simulink model "Dynamics"  (R2015a)
settings: Solver=ode45  StartTime=0.0  StopTime=50  FixedStep=1e-3
libraries: aerolibutil x16, aerolibtransform2 x6, dspmtrx3 x6
(part 2 of 2)

== system Dynamics/Jacobian/J_v/J_v_3 ==
  R : Inport
  p : Inport  Port=2
  pn : Inport  Port=3
  type : Inport  Port=4
  Add : Sum
  If : If  IfExpression=u1 == 1
  Prismatic Action : Subsystem  TreatAsAtomicUnit=on
  Revolute Action : Subsystem  TreatAsAtomicUnit=on
  J_v : Outport
  wires:
  type/1 -> If/1
  If/1 -> Revolute Action/Action
  If/2 -> Prismatic Action/Action
  Revolute Action/1(J_v) -> Add/1
  Prismatic Action/1(J_v) -> Add/2
  Add/1 -> J_v/1
  R/1 -> Prismatic Action/1(R), Revolute Action/1(R)
  p/1 -> Revolute Action/2(p)
  pn/1 -> Revolute Action/3(pn)

== system Dynamics/Jacobian/J_v/J_v_4 ==
  R : Inport
  p : Inport  Port=2
  pn : Inport  Port=3
  type : Inport  Port=4
  Add : Sum
  If : If  IfExpression=u1 == 1
  Prismatic Action : Subsystem  TreatAsAtomicUnit=on
  Revolute Action : Subsystem  TreatAsAtomicUnit=on
  J_v : Outport
  wires:
  type/1 -> If/1
  If/1 -> Revolute Action/Action
  If/2 -> Prismatic Action/Action
  Revolute Action/1(J_v) -> Add/1
  Prismatic Action/1(J_v) -> Add/2
  Add/1 -> J_v/1
  R/1 -> Prismatic Action/1(R), Revolute Action/1(R)
  p/1 -> Revolute Action/2(p)
  pn/1 -> Revolute Action/3(pn)

== system Dynamics/Jacobian/J_v/J_v_5 ==
  R : Inport
  p : Inport  Port=2
  pn : Inport  Port=3
  type : Inport  Port=4
  Add : Sum
  If : If  IfExpression=u1 == 1
  Prismatic Action : Subsystem  TreatAsAtomicUnit=on
  Revolute Action : Subsystem  TreatAsAtomicUnit=on
  J_v : Outport
  wires:
  type/1 -> If/1
  If/1 -> Revolute Action/Action
  If/2 -> Prismatic Action/Action
  Revolute Action/1(J_v) -> Add/1
  Prismatic Action/1(J_v) -> Add/2
  Add/1 -> J_v/1
  R/1 -> Prismatic Action/1(R), Revolute Action/1(R)
  p/1 -> Revolute Action/2(p)
  pn/1 -> Revolute Action/3(pn)

== system Dynamics/Jacobian/J_v/J_v_6 ==
  R : Inport
  p : Inport  Port=2
  pn : Inport  Port=3
  type : Inport  Port=4
  Add : Sum
  If : If  IfExpression=u1 == 1
  Prismatic Action : Subsystem  TreatAsAtomicUnit=on
  Revolute Action : Subsystem  TreatAsAtomicUnit=on
  J_v : Outport
  wires:
  type/1 -> If/1
  If/1 -> Revolute Action/Action
  If/2 -> Prismatic Action/Action
  Revolute Action/1(J_v) -> Add/1
  Prismatic Action/1(J_v) -> Add/2
  Add/1 -> J_v/1
  R/1 -> Prismatic Action/1(R), Revolute Action/1(R)
  p/1 -> Revolute Action/2(p)
  pn/1 -> Revolute Action/3(pn)

== system Dynamics/Jacobian/J(q) gen./J_v_2(q)/J_v_1 ==
  R : Inport
  p : Inport  Port=2
  pn : Inport  Port=3
  type : Inport  Port=4
  Add : Sum
  If : If  IfExpression=u1 == 1
  Prismatic Action : Subsystem  TreatAsAtomicUnit=on
  Revolute Action : Subsystem  TreatAsAtomicUnit=on
  J_v : Outport
  wires:
  type/1 -> If/1
  If/1 -> Revolute Action/Action
  If/2 -> Prismatic Action/Action
  Revolute Action/1(J_v) -> Add/1
  Prismatic Action/1(J_v) -> Add/2
  Add/1 -> J_v/1
  R/1 -> Prismatic Action/1(R), Revolute Action/1(R)
  p/1 -> Revolute Action/2(p)
  pn/1 -> Revolute Action/3(pn)

== system Dynamics/Jacobian/J(q) gen./J_v_3(q)/J_v_1 ==
  R : Inport
  p : Inport  Port=2
  pn : Inport  Port=3
  type : Inport  Port=4
  Add : Sum
  If : If  IfExpression=u1 == 1
  Prismatic Action : Subsystem  TreatAsAtomicUnit=on
  Revolute Action : Subsystem  TreatAsAtomicUnit=on
  J_v : Outport
  wires:
  type/1 -> If/1
  If/1 -> Revolute Action/Action
  If/2 -> Prismatic Action/Action
  Revolute Action/1(J_v) -> Add/1
  Prismatic Action/1(J_v) -> Add/2
  Add/1 -> J_v/1
  R/1 -> Prismatic Action/1(R), Revolute Action/1(R)
  p/1 -> Revolute Action/2(p)
  pn/1 -> Revolute Action/3(pn)

== system Dynamics/Jacobian/J(q) gen./J_v_3(q)/J_v_2 ==
  R : Inport
  p : Inport  Port=2
  pn : Inport  Port=3
  type : Inport  Port=4
  Add : Sum
  If : If  IfExpression=u1 == 1
  Prismatic Action : Subsystem  TreatAsAtomicUnit=on
  Revolute Action : Subsystem  TreatAsAtomicUnit=on
  J_v : Outport
  wires:
  type/1 -> If/1
  If/1 -> Revolute Action/Action
  If/2 -> Prismatic Action/Action
  Revolute Action/1(J_v) -> Add/1
  Prismatic Action/1(J_v) -> Add/2
  Add/1 -> J_v/1
  R/1 -> Prismatic Action/1(R), Revolute Action/1(R)
  p/1 -> Revolute Action/2(p)
  pn/1 -> Revolute Action/3(pn)

== system Dynamics/Jacobian/J(q) gen./J_v_4(q)/J_v_1 ==
  R : Inport
  p : Inport  Port=2
  pn : Inport  Port=3
  type : Inport  Port=4
  Add : Sum
  If : If  IfExpression=u1 == 1
  Prismatic Action : Subsystem  TreatAsAtomicUnit=on
  Revolute Action : Subsystem  TreatAsAtomicUnit=on
  J_v : Outport
  wires:
  type/1 -> If/1
  If/1 -> Revolute Action/Action
  If/2 -> Prismatic Action/Action
  Revolute Action/1(J_v) -> Add/1
  Prismatic Action/1(J_v) -> Add/2
  Add/1 -> J_v/1
  R/1 -> Prismatic Action/1(R), Revolute Action/1(R)
  p/1 -> Revolute Action/2(p)
  pn/1 -> Revolute Action/3(pn)

== system Dynamics/Jacobian/J(q) gen./J_v_4(q)/J_v_2 ==
  R : Inport
  p : Inport  Port=2
  pn : Inport  Port=3
  type : Inport  Port=4
  Add : Sum
  If : If  IfExpression=u1 == 1
  Prismatic Action : Subsystem  TreatAsAtomicUnit=on
  Revolute Action : Subsystem  TreatAsAtomicUnit=on
  J_v : Outport
  wires:
  type/1 -> If/1
  If/1 -> Revolute Action/Action
  If/2 -> Prismatic Action/Action
  Revolute Action/1(J_v) -> Add/1
  Prismatic Action/1(J_v) -> Add/2
  Add/1 -> J_v/1
  R/1 -> Prismatic Action/1(R), Revolute Action/1(R)
  p/1 -> Revolute Action/2(p)
  pn/1 -> Revolute Action/3(pn)

== system Dynamics/Jacobian/J(q) gen./J_v_4(q)/J_v_3 ==
  R : Inport
  p : Inport  Port=2
  pn : Inport  Port=3
  type : Inport  Port=4
  Add : Sum
  If : If  IfExpression=u1 == 1
  Prismatic Action : Subsystem  TreatAsAtomicUnit=on
  Revolute Action : Subsystem  TreatAsAtomicUnit=on
  J_v : Outport
  wires:
  type/1 -> If/1
  If/1 -> Revolute Action/Action
  If/2 -> Prismatic Action/Action
  Revolute Action/1(J_v) -> Add/1
  Prismatic Action/1(J_v) -> Add/2
  Add/1 -> J_v/1
  R/1 -> Prismatic Action/1(R), Revolute Action/1(R)
  p/1 -> Revolute Action/2(p)
  pn/1 -> Revolute Action/3(pn)

== system Dynamics/Jacobian/J(q) gen./J_v_5(q)/J_v_1 ==
  R : Inport
  p : Inport  Port=2
  pn : Inport  Port=3
  type : Inport  Port=4
  Add : Sum
  If : If  IfExpression=u1 == 1
  Prismatic Action : Subsystem  TreatAsAtomicUnit=on
  Revolute Action : Subsystem  TreatAsAtomicUnit=on
  J_v : Outport
  wires:
  type/1 -> If/1
  If/1 -> Revolute Action/Action
  If/2 -> Prismatic Action/Action
  Revolute Action/1(J_v) -> Add/1
  Prismatic Action/1(J_v) -> Add/2
  Add/1 -> J_v/1
  R/1 -> Prismatic Action/1(R), Revolute Action/1(R)
  p/1 -> Revolute Action/2(p)
  pn/1 -> Revolute Action/3(pn)

== system Dynamics/Jacobian/J(q) gen./J_v_5(q)/J_v_2 ==
  R : Inport
  p : Inport  Port=2
  pn : Inport  Port=3
  type : Inport  Port=4
  Add : Sum
  If : If  IfExpression=u1 == 1
  Prismatic Action : Subsystem  TreatAsAtomicUnit=on
  Revolute Action : Subsystem  TreatAsAtomicUnit=on
  J_v : Outport
  wires:
  type/1 -> If/1
  If/1 -> Revolute Action/Action
  If/2 -> Prismatic Action/Action
  Revolute Action/1(J_v) -> Add/1
  Prismatic Action/1(J_v) -> Add/2
  Add/1 -> J_v/1
  R/1 -> Prismatic Action/1(R), Revolute Action/1(R)
  p/1 -> Revolute Action/2(p)
  pn/1 -> Revolute Action/3(pn)

== system Dynamics/Jacobian/J(q) gen./J_v_5(q)/J_v_3 ==
  R : Inport
  p : Inport  Port=2
  pn : Inport  Port=3
  type : Inport  Port=4
  Add : Sum
  If : If  IfExpression=u1 == 1
  Prismatic Action : Subsystem  TreatAsAtomicUnit=on
  Revolute Action : Subsystem  TreatAsAtomicUnit=on
  J_v : Outport
  wires:
  type/1 -> If/1
  If/1 -> Revolute Action/Action
  If/2 -> Prismatic Action/Action
  Revolute Action/1(J_v) -> Add/1
  Prismatic Action/1(J_v) -> Add/2
  Add/1 -> J_v/1
  R/1 -> Prismatic Action/1(R), Revolute Action/1(R)
  p/1 -> Revolute Action/2(p)
  pn/1 -> Revolute Action/3(pn)

== system Dynamics/Jacobian/J(q) gen./J_v_5(q)/J_v_4 ==
  R : Inport
  p : Inport  Port=2
  pn : Inport  Port=3
  type : Inport  Port=4
  Add : Sum
  If : If  IfExpression=u1 == 1
  Prismatic Action : Subsystem  TreatAsAtomicUnit=on
  Revolute Action : Subsystem  TreatAsAtomicUnit=on
  J_v : Outport
  wires:
  type/1 -> If/1
  If/1 -> Revolute Action/Action
  If/2 -> Prismatic Action/Action
  Revolute Action/1(J_v) -> Add/1
  Prismatic Action/1(J_v) -> Add/2
  Add/1 -> J_v/1
  R/1 -> Prismatic Action/1(R), Revolute Action/1(R)
  p/1 -> Revolute Action/2(p)
  pn/1 -> Revolute Action/3(pn)

== system Dynamics/Jacobian/J_v/J_v_1/Prismatic Action ==
  R : Inport
  Action Port : ActionPort  ActionType=else
  Constant : Constant  Value=[0;0;1]
  Product : Product  Multiplication=Matrix(*)
  J_v : Outport
  wires:
  Product/1 -> J_v/1
  R/1 -> Product/1
  Constant/1 -> Product/2

== system Dynamics/Jacobian/J_v/J_v_1/Revolute Action ==
  R : Inport
  p : Inport  Port=2
  pn : Inport  Port=3
  Action Port : ActionPort  ActionType=then
  3x3 Cross Product : aerolibutil/3x3 Cross Product
  Add : Sum  Inputs=-+
  Constant : Constant  Value=[0;0;1]
  Product : Product  Multiplication=Matrix(*)
  J_v : Outport
  wires:
  3x3 Cross Product/1 -> J_v/1
  p/1 -> Add/1
  pn/1 -> Add/2
  Add/1 -> 3x3 Cross Product/2
  R/1 -> Product/1
  Constant/1 -> Product/2
  Product/1 -> 3x3 Cross Product/1

== system Dynamics/Jacobian/J_v/J_v_2/Prismatic Action ==
  R : Inport
  Action Port : ActionPort  ActionType=else
  Constant : Constant  Value=[0;0;1]
  Product : Product  Multiplication=Matrix(*)
  J_v : Outport
  wires:
  Product/1 -> J_v/1
  R/1 -> Product/1
  Constant/1 -> Product/2

== system Dynamics/Jacobian/J_v/J_v_2/Revolute Action ==
  R : Inport
  p : Inport  Port=2
  pn : Inport  Port=3
  Action Port : ActionPort  ActionType=then
  3x3 Cross Product : aerolibutil/3x3 Cross Product
  Add : Sum  Inputs=-+
  Constant : Constant  Value=[0;0;1]
  Product : Product  Multiplication=Matrix(*)
  J_v : Outport
  wires:
  3x3 Cross Product/1 -> J_v/1
  p/1 -> Add/1
  pn/1 -> Add/2
  Add/1 -> 3x3 Cross Product/2
  R/1 -> Product/1
  Constant/1 -> Product/2
  Product/1 -> 3x3 Cross Product/1

== system Dynamics/Jacobian/J_v/J_v_3/Prismatic Action ==
  R : Inport
  Action Port : ActionPort  ActionType=else
  Constant : Constant  Value=[0;0;1]
  Product : Product  Multiplication=Matrix(*)
  J_v : Outport
  wires:
  Product/1 -> J_v/1
  R/1 -> Product/1
  Constant/1 -> Product/2

== system Dynamics/Jacobian/J_v/J_v_3/Revolute Action ==
  R : Inport
  p : Inport  Port=2
  pn : Inport  Port=3
  Action Port : ActionPort  ActionType=then
  3x3 Cross Product : aerolibutil/3x3 Cross Product
  Add : Sum  Inputs=-+
  Constant : Constant  Value=[0;0;1]
  Product : Product  Multiplication=Matrix(*)
  J_v : Outport
  wires:
  3x3 Cross Product/1 -> J_v/1
  p/1 -> Add/1
  pn/1 -> Add/2
  Add/1 -> 3x3 Cross Product/2
  R/1 -> Product/1
  Constant/1 -> Product/2
  Product/1 -> 3x3 Cross Product/1

== system Dynamics/Jacobian/J_v/J_v_4/Prismatic Action ==
  R : Inport
  Action Port : ActionPort  ActionType=else
  Constant : Constant  Value=[0;0;1]
  Product : Product  Multiplication=Matrix(*)
  J_v : Outport
  wires:
  Product/1 -> J_v/1
  R/1 -> Product/1
  Constant/1 -> Product/2

== system Dynamics/Jacobian/J_v/J_v_4/Revolute Action ==
  R : Inport
  p : Inport  Port=2
  pn : Inport  Port=3
  Action Port : ActionPort  ActionType=then
  3x3 Cross Product : aerolibutil/3x3 Cross Product
  Add : Sum  Inputs=-+
  Constant : Constant  Value=[0;0;1]
  Product : Product  Multiplication=Matrix(*)
  J_v : Outport
  wires:
  3x3 Cross Product/1 -> J_v/1
  p/1 -> Add/1
  pn/1 -> Add/2
  Add/1 -> 3x3 Cross Product/2
  R/1 -> Product/1
  Constant/1 -> Product/2
  Product/1 -> 3x3 Cross Product/1

== system Dynamics/Jacobian/J_v/J_v_5/Prismatic Action ==
  R : Inport
  Action Port : ActionPort  ActionType=else
  Constant : Constant  Value=[0;0;1]
  Product : Product  Multiplication=Matrix(*)
  J_v : Outport
  wires:
  Product/1 -> J_v/1
  R/1 -> Product/1
  Constant/1 -> Product/2

== system Dynamics/Jacobian/J_v/J_v_5/Revolute Action ==
  R : Inport
  p : Inport  Port=2
  pn : Inport  Port=3
  Action Port : ActionPort  ActionType=then
  3x3 Cross Product : aerolibutil/3x3 Cross Product
  Add : Sum  Inputs=-+
  Constant : Constant  Value=[0;0;1]
  Product : Product  Multiplication=Matrix(*)
  J_v : Outport
  wires:
  3x3 Cross Product/1 -> J_v/1
  p/1 -> Add/1
  pn/1 -> Add/2
  Add/1 -> 3x3 Cross Product/2
  R/1 -> Product/1
  Constant/1 -> Product/2
  Product/1 -> 3x3 Cross Product/1

== system Dynamics/Jacobian/J_v/J_v_6/Prismatic Action ==
  R : Inport
  Action Port : ActionPort  ActionType=else
  Constant : Constant  Value=[0;0;1]
  Product : Product  Multiplication=Matrix(*)
  J_v : Outport
  wires:
  Product/1 -> J_v/1
  R/1 -> Product/1
  Constant/1 -> Product/2

== system Dynamics/Jacobian/J_v/J_v_6/Revolute Action ==
  R : Inport
  p : Inport  Port=2
  pn : Inport  Port=3
  Action Port : ActionPort  ActionType=then
  3x3 Cross Product : aerolibutil/3x3 Cross Product
  Add : Sum  Inputs=-+
  Constant : Constant  Value=[0;0;1]
  Product : Product  Multiplication=Matrix(*)
  J_v : Outport
  wires:
  3x3 Cross Product/1 -> J_v/1
  p/1 -> Add/1
  pn/1 -> Add/2
  Add/1 -> 3x3 Cross Product/2
  R/1 -> Product/1
  Constant/1 -> Product/2
  Product/1 -> 3x3 Cross Product/1

== system Dynamics/Jacobian/J(q) gen./J_v_2(q)/J_v_1/Prismatic Action ==
  R : Inport
  Action Port : ActionPort  ActionType=else
  Constant : Constant  Value=[0;0;1]
  Product : Product  Multiplication=Matrix(*)
  J_v : Outport
  wires:
  Product/1 -> J_v/1
  R/1 -> Product/1
  Constant/1 -> Product/2

== system Dynamics/Jacobian/J(q) gen./J_v_2(q)/J_v_1/Revolute Action ==
  R : Inport
  p : Inport  Port=2
  pn : Inport  Port=3
  Action Port : ActionPort  ActionType=then
  3x3 Cross Product : aerolibutil/3x3 Cross Product
  Add : Sum  Inputs=-+
  Constant : Constant  Value=[0;0;1]
  Product : Product  Multiplication=Matrix(*)
  J_v : Outport
  wires:
  3x3 Cross Product/1 -> J_v/1
  p/1 -> Add/1
  pn/1 -> Add/2
  Add/1 -> 3x3 Cross Product/2
  R/1 -> Product/1
  Constant/1 -> Product/2
  Product/1 -> 3x3 Cross Product/1

== system Dynamics/Jacobian/J(q) gen./J_v_3(q)/J_v_1/Prismatic Action ==
  R : Inport
  Action Port : ActionPort  ActionType=else
  Constant : Constant  Value=[0;0;1]
  Product : Product  Multiplication=Matrix(*)
  J_v : Outport
  wires:
  Product/1 -> J_v/1
  R/1 -> Product/1
  Constant/1 -> Product/2

== system Dynamics/Jacobian/J(q) gen./J_v_3(q)/J_v_1/Revolute Action ==
  R : Inport
  p : Inport  Port=2
  pn : Inport  Port=3
  Action Port : ActionPort  ActionType=then
  3x3 Cross Product : aerolibutil/3x3 Cross Product
  Add : Sum  Inputs=-+
  Constant : Constant  Value=[0;0;1]
  Product : Product  Multiplication=Matrix(*)
  J_v : Outport
  wires:
  3x3 Cross Product/1 -> J_v/1
  p/1 -> Add/1
  pn/1 -> Add/2
  Add/1 -> 3x3 Cross Product/2
  R/1 -> Product/1
  Constant/1 -> Product/2
  Product/1 -> 3x3 Cross Product/1

== system Dynamics/Jacobian/J(q) gen./J_v_3(q)/J_v_2/Prismatic Action ==
  R : Inport
  Action Port : ActionPort  ActionType=else
  Constant : Constant  Value=[0;0;1]
  Product : Product  Multiplication=Matrix(*)
  J_v : Outport
  wires:
  Product/1 -> J_v/1
  R/1 -> Product/1
  Constant/1 -> Product/2

== system Dynamics/Jacobian/J(q) gen./J_v_3(q)/J_v_2/Revolute Action ==
  R : Inport
  p : Inport  Port=2
  pn : Inport  Port=3
  Action Port : ActionPort  ActionType=then
  3x3 Cross Product : aerolibutil/3x3 Cross Product
  Add : Sum  Inputs=-+
  Constant : Constant  Value=[0;0;1]
  Product : Product  Multiplication=Matrix(*)
  J_v : Outport
  wires:
  3x3 Cross Product/1 -> J_v/1
  p/1 -> Add/1
  pn/1 -> Add/2
  Add/1 -> 3x3 Cross Product/2
  R/1 -> Product/1
  Constant/1 -> Product/2
  Product/1 -> 3x3 Cross Product/1

== system Dynamics/Jacobian/J(q) gen./J_v_4(q)/J_v_1/Prismatic Action ==
  R : Inport
  Action Port : ActionPort  ActionType=else
  Constant : Constant  Value=[0;0;1]
  Product : Product  Multiplication=Matrix(*)
  J_v : Outport
  wires:
  Product/1 -> J_v/1
  R/1 -> Product/1
  Constant/1 -> Product/2

== system Dynamics/Jacobian/J(q) gen./J_v_4(q)/J_v_1/Revolute Action ==
  R : Inport
  p : Inport  Port=2
  pn : Inport  Port=3
  Action Port : ActionPort  ActionType=then
  3x3 Cross Product : aerolibutil/3x3 Cross Product
  Add : Sum  Inputs=-+
  Constant : Constant  Value=[0;0;1]
  Product : Product  Multiplication=Matrix(*)
  J_v : Outport
  wires:
  3x3 Cross Product/1 -> J_v/1
  p/1 -> Add/1
  pn/1 -> Add/2
  Add/1 -> 3x3 Cross Product/2
  R/1 -> Product/1
  Constant/1 -> Product/2
  Product/1 -> 3x3 Cross Product/1

== system Dynamics/Jacobian/J(q) gen./J_v_4(q)/J_v_2/Prismatic Action ==
  R : Inport
  Action Port : ActionPort  ActionType=else
  Constant : Constant  Value=[0;0;1]
  Product : Product  Multiplication=Matrix(*)
  J_v : Outport
  wires:
  Product/1 -> J_v/1
  R/1 -> Product/1
  Constant/1 -> Product/2

== system Dynamics/Jacobian/J(q) gen./J_v_4(q)/J_v_2/Revolute Action ==
  R : Inport
  p : Inport  Port=2
  pn : Inport  Port=3
  Action Port : ActionPort  ActionType=then
  3x3 Cross Product : aerolibutil/3x3 Cross Product
  Add : Sum  Inputs=-+
  Constant : Constant  Value=[0;0;1]
  Product : Product  Multiplication=Matrix(*)
  J_v : Outport
  wires:
  3x3 Cross Product/1 -> J_v/1
  p/1 -> Add/1
  pn/1 -> Add/2
  Add/1 -> 3x3 Cross Product/2
  R/1 -> Product/1
  Constant/1 -> Product/2
  Product/1 -> 3x3 Cross Product/1

== system Dynamics/Jacobian/J(q) gen./J_v_4(q)/J_v_3/Prismatic Action ==
  R : Inport
  Action Port : ActionPort  ActionType=else
  Constant : Constant  Value=[0;0;1]
  Product : Product  Multiplication=Matrix(*)
  J_v : Outport
  wires:
  Product/1 -> J_v/1
  R/1 -> Product/1
  Constant/1 -> Product/2

== system Dynamics/Jacobian/J(q) gen./J_v_4(q)/J_v_3/Revolute Action ==
  R : Inport
  p : Inport  Port=2
  pn : Inport  Port=3
  Action Port : ActionPort  ActionType=then
  3x3 Cross Product : aerolibutil/3x3 Cross Product
  Add : Sum  Inputs=-+
  Constant : Constant  Value=[0;0;1]
  Product : Product  Multiplication=Matrix(*)
  J_v : Outport
  wires:
  3x3 Cross Product/1 -> J_v/1
  p/1 -> Add/1
  pn/1 -> Add/2
  Add/1 -> 3x3 Cross Product/2
  R/1 -> Product/1
  Constant/1 -> Product/2
  Product/1 -> 3x3 Cross Product/1

== system Dynamics/Jacobian/J(q) gen./J_v_5(q)/J_v_1/Prismatic Action ==
  R : Inport
  Action Port : ActionPort  ActionType=else
  Constant : Constant  Value=[0;0;1]
  Product : Product  Multiplication=Matrix(*)
  J_v : Outport
  wires:
  Product/1 -> J_v/1
  R/1 -> Product/1
  Constant/1 -> Product/2

== system Dynamics/Jacobian/J(q) gen./J_v_5(q)/J_v_1/Revolute Action ==
  R : Inport
  p : Inport  Port=2
  pn : Inport  Port=3
  Action Port : ActionPort  ActionType=then
  3x3 Cross Product : aerolibutil/3x3 Cross Product
  Add : Sum  Inputs=-+
  Constant : Constant  Value=[0;0;1]
  Product : Product  Multiplication=Matrix(*)
  J_v : Outport
  wires:
  3x3 Cross Product/1 -> J_v/1
  p/1 -> Add/1
  pn/1 -> Add/2
  Add/1 -> 3x3 Cross Product/2
  R/1 -> Product/1
  Constant/1 -> Product/2
  Product/1 -> 3x3 Cross Product/1

== system Dynamics/Jacobian/J(q) gen./J_v_5(q)/J_v_2/Prismatic Action ==
  R : Inport
  Action Port : ActionPort  ActionType=else
  Constant : Constant  Value=[0;0;1]
  Product : Product  Multiplication=Matrix(*)
  J_v : Outport
  wires:
  Product/1 -> J_v/1
  R/1 -> Product/1
  Constant/1 -> Product/2

== system Dynamics/Jacobian/J(q) gen./J_v_5(q)/J_v_2/Revolute Action ==
  R : Inport
  p : Inport  Port=2
  pn : Inport  Port=3
  Action Port : ActionPort  ActionType=then
  3x3 Cross Product : aerolibutil/3x3 Cross Product
  Add : Sum  Inputs=-+
  Constant : Constant  Value=[0;0;1]
  Product : Product  Multiplication=Matrix(*)
  J_v : Outport
  wires:
  3x3 Cross Product/1 -> J_v/1
  p/1 -> Add/1
  pn/1 -> Add/2
  Add/1 -> 3x3 Cross Product/2
  R/1 -> Product/1
  Constant/1 -> Product/2
  Product/1 -> 3x3 Cross Product/1

== system Dynamics/Jacobian/J(q) gen./J_v_5(q)/J_v_3/Prismatic Action ==
  R : Inport
  Action Port : ActionPort  ActionType=else
  Constant : Constant  Value=[0;0;1]
  Product : Product  Multiplication=Matrix(*)
  J_v : Outport
  wires:
  Product/1 -> J_v/1
  R/1 -> Product/1
  Constant/1 -> Product/2

== system Dynamics/Jacobian/J(q) gen./J_v_5(q)/J_v_3/Revolute Action ==
  R : Inport
  p : Inport  Port=2
  pn : Inport  Port=3
  Action Port : ActionPort  ActionType=then
  3x3 Cross Product : aerolibutil/3x3 Cross Product
  Add : Sum  Inputs=-+
  Constant : Constant  Value=[0;0;1]
  Product : Product  Multiplication=Matrix(*)
  J_v : Outport
  wires:
  3x3 Cross Product/1 -> J_v/1
  p/1 -> Add/1
  pn/1 -> Add/2
  Add/1 -> 3x3 Cross Product/2
  R/1 -> Product/1
  Constant/1 -> Product/2
  Product/1 -> 3x3 Cross Product/1

== system Dynamics/Jacobian/J(q) gen./J_v_5(q)/J_v_4/Prismatic Action ==
  R : Inport
  Action Port : ActionPort  ActionType=else
  Constant : Constant  Value=[0;0;1]
  Product : Product  Multiplication=Matrix(*)
  J_v : Outport
  wires:
  Product/1 -> J_v/1
  R/1 -> Product/1
  Constant/1 -> Product/2

== system Dynamics/Jacobian/J(q) gen./J_v_5(q)/J_v_4/Revolute Action ==
  R : Inport
  p : Inport  Port=2
  pn : Inport  Port=3
  Action Port : ActionPort  ActionType=then
  3x3 Cross Product : aerolibutil/3x3 Cross Product
  Add : Sum  Inputs=-+
  Constant : Constant  Value=[0;0;1]
  Product : Product  Multiplication=Matrix(*)
  J_v : Outport
  wires:
  3x3 Cross Product/1 -> J_v/1
  p/1 -> Add/1
  pn/1 -> Add/2
  Add/1 -> 3x3 Cross Product/2
  R/1 -> Product/1
  Constant/1 -> Product/2
  Product/1 -> 3x3 Cross Product/1

== matlab function Dynamics/H_6^0/H_5^4/MATLAB Function ==
  data: R input; H output; p input
function H = fcn(R,p)

H = [R          p
     zeros(1,3) 1];

== matlab function Dynamics/H_6^0/H_4^3/MATLAB Function ==
  data: R input; H output; p input
function H = fcn(R,p)

H = [R          p
     zeros(1,3) 1];

== matlab function Dynamics/H_6^0/H_3^2/MATLAB Function ==
  data: R input; H output; p input
function H = fcn(R,p)

H = [R          p
     zeros(1,3) 1];

== matlab function Dynamics/H_6^0/H_2^1/MATLAB Function ==
  data: R input; H output; p input
function H = fcn(R,p)

H = [R          p
     zeros(1,3) 1];

== matlab function Dynamics/H_6^0/H_1^0/MATLAB Function ==
  data: R input; H output; p input
function H = fcn(R,p)

H = [R          p
     zeros(1,3) 1];

== matlab function Dynamics/Jacobian/J(q) gen./J_v_1(q)/v2M_1 ==
  data: v1 input; M output; v2 input
function M = fcn(v1,v2)

M=[v1 v2];

== matlab function Dynamics/Jacobian/J_w/J_w_1 ==
  data: R input; J_w output; type input
function J_w = fcn(R,type)

if type==1
    
    J_w=R*[0;0;1];
    
else
    
    J_w=zeros(3,1);
    
end

== matlab function Dynamics/H_6^0/H_6^5/MATLAB Function ==
  data: R input; H output; p input
function H = fcn(R,p)

H = [R          p
     zeros(1,3) 1];

== matlab function Dynamics/Jacobian/J_w/J_w_2 ==
  data: R input; J_w output; type input
function J_w = fcn(R,type)

if type==1
    
    J_w=R*[0;0;1];
    
else
    
    J_w=zeros(3,1);
    
end

== matlab function Dynamics/Jacobian/J_w/J_w_3 ==
  data: R input; J_w output; type input
function J_w = fcn(R,type)

if type==1
    
    J_w=R*[0;0;1];
    
else
    
    J_w=zeros(3,1);
    
end

== matlab function Dynamics/Jacobian/J_w/J_w_4 ==
  data: R input; J_w output; type input
function J_w = fcn(R,type)

if type==1
    
    J_w=R*[0;0;1];
    
else
    
    J_w=zeros(3,1);
    
end

== matlab function Dynamics/Jacobian/J_w/J_w_5 ==
  data: R input; J_w output; type input
function J_w = fcn(R,type)

if type==1
    
    J_w=R*[0;0;1];
    
else
    
    J_w=zeros(3,1);
    
end

== matlab function Dynamics/Jacobian/J_w/J_w_6 ==
  data: R input; J_w output; type input
function J_w = fcn(R,type)

if type==1
    
    J_w=R*[0;0;1];
    
else
    
    J_w=zeros(3,1);
    
end

== matlab function Dynamics/Jacobian/J_w/v2M_1 ==
  data: v1 input; M output; v2 input
function M = fcn(v1,v2)

M=[v1 v2];

== matlab function Dynamics/Jacobian/J_w/v2M_2 ==
  data: v1 input; M output; v2 input
function M = fcn(v1,v2)

M=[v1 v2];

== matlab function Dynamics/Jacobian/J_w/v2M_3 ==
  data: v1 input; M output; v2 input
function M = fcn(v1,v2)

M=[v1 v2];

== matlab function Dynamics/Jacobian/J_w/v2M_4 ==
  data: v1 input; M output; v2 input
function M = fcn(v1,v2)

M=[v1 v2];

== matlab function Dynamics/Jacobian/J_w/v2M_5 ==
  data: v1 input; M output; v2 input
function M = fcn(v1,v2)

M=[v1 v2];

== matlab function Dynamics/Jacobian/J(q) gen./J_v_1(q)/v2M_2 ==
  data: v1 input; M output; v2 input
function M = fcn(v1,v2)

M=[v1 v2];

== matlab function Dynamics/Jacobian/J(q) gen./J_v_1(q)/v2M_3 ==
  data: v1 input; M output; v2 input
function M = fcn(v1,v2)

M=[v1 v2];

== matlab function Dynamics/Jacobian/J(q) gen./J_v_1(q)/v2M_4 ==
  data: v1 input; M output; v2 input
function M = fcn(v1,v2)

M=[v1 v2];

== matlab function Dynamics/Jacobian/J(q) gen./J_v_1(q)/v2M_5 ==
  data: v1 input; M output; v2 input
function M = fcn(v1,v2)

M=[v1 v2];

== matlab function Dynamics/Jacobian/J(q) gen./J_v_2(q)/v2M_1 ==
  data: v1 input; M output; v2 input
function M = fcn(v1,v2)

M=[v1 v2];

== matlab function Dynamics/Jacobian/J(q) gen./J_v_2(q)/v2M_2 ==
  data: v1 input; M output; v2 input
function M = fcn(v1,v2)

M=[v1 v2];

== matlab function Dynamics/Jacobian/J_v/v2M_1 ==
  data: v1 input; M output; v2 input
function M = fcn(v1,v2)

M=[v1 v2];

== matlab function Dynamics/Jacobian/J_v/v2M_2 ==
  data: v1 input; M output; v2 input
function M = fcn(v1,v2)

M=[v1 v2];

== matlab function Dynamics/Jacobian/J_v/v2M_3 ==
  data: v1 input; M output; v2 input
function M = fcn(v1,v2)

M=[v1 v2];

== matlab function Dynamics/Jacobian/J_v/v2M_4 ==
  data: v1 input; M output; v2 input
function M = fcn(v1,v2)

M=[v1 v2];

== matlab function Dynamics/Jacobian/J_v/v2M_5 ==
  data: v1 input; M output; v2 input
function M = fcn(v1,v2)

M=[v1 v2];

== matlab function Dynamics/M(q),C(q,dq),g(q)/M,H/MATLAB Function ==
  data: m input; M output; I1 input; I2 input; I3 input; I4 input; I5 input; I6 input; W1 input; W2 input; W3 input; W4 input; W5 input; W6 input; H output
function [M,H] = fcn(m,I1,I2,I3,I4,I5,I6,W1,W2,W3,W4,W5,W6)
%#codegen

M = blkdiag(m(1)*eye(3),m(2)*eye(3),m(3)*eye(3),m(4)*eye(3),m(5)*eye(3),m(6)*eye(3),...
            I1,I2,I3,I4,I5,I6);

H =-blkdiag(zeros(18,18),W1,W2,W3,W4,W5,W6);

== matlab function Dynamics/M(q),C(q,dq),g(q)/M,H/W1 ==
  data: w1 input; W output; w2 input; w3 input
function W = fcn(w1,w2,w3)

W = [0    -w3  w2
     w3    0  -w1
    -w2    w1  0];

== matlab function Dynamics/M(q),C(q,dq),g(q)/M,H/W2 ==
  data: w1 input; W output; w2 input; w3 input
function W = fcn(w1,w2,w3)

W = [0    -w3  w2
     w3  0    -w1
    -w2  w1  0];

== matlab function Dynamics/M(q),C(q,dq),g(q)/M,H/W3 ==
  data: w1 input; W output; w2 input; w3 input
function W = fcn(w1,w2,w3)

W = [0    -w3  w2
     w3  0    -w1
    -w2  w1  0];

== matlab function Dynamics/M(q),C(q,dq),g(q)/M,H/W4 ==
  data: w1 input; W output; w2 input; w3 input
function W = fcn(w1,w2,w3)

W = [0    -w3  w2
     w3  0    -w1
    -w2  w1  0];

== matlab function Dynamics/M(q),C(q,dq),g(q)/M,H/W5 ==
  data: w1 input; W output; w2 input; w3 input
function W = fcn(w1,w2,w3)

W = [0    -w3  w2
     w3  0    -w1
    -w2  w1  0];

== matlab function Dynamics/M(q),C(q,dq),g(q)/M,H/W6 ==
  data: w1 input; W output; w2 input; w3 input
function W = fcn(w1,w2,w3)

W = [0    -w3  w2
     w3  0    -w1
    -w2  w1  0];

== matlab function Dynamics/Jacobian/J(q) gen./J_v_2(q)/v2M_3 ==
  data: v1 input; M output; v2 input
function M = fcn(v1,v2)

M=[v1 v2];

== matlab function Dynamics/Jacobian/J(q) gen./J_v_2(q)/v2M_4 ==
  data: v1 input; M output; v2 input
function M = fcn(v1,v2)

M=[v1 v2];

== matlab function Dynamics/Jacobian/J(q) gen./J_v_2(q)/v2M_5 ==
  data: v1 input; M output; v2 input
function M = fcn(v1,v2)

M=[v1 v2];

== matlab function Dynamics/Jacobian/J(q) gen./J_v_3(q)/v2M_1 ==
  data: v1 input; M output; v2 input
function M = fcn(v1,v2)

M=[v1 v2];

== matlab function Dynamics/Jacobian/J(q) gen./J_v_3(q)/v2M_2 ==
  data: v1 input; M output; v2 input
function M = fcn(v1,v2)

M=[v1 v2];

== matlab function Dynamics/Jacobian/J(q) gen./J_v_3(q)/v2M_3 ==
  data: v1 input; M output; v2 input
function M = fcn(v1,v2)

M=[v1 v2];

== matlab function Dynamics/Jacobian/J(q) gen./J_v_3(q)/v2M_4 ==
  data: v1 input; M output; v2 input
function M = fcn(v1,v2)

M=[v1 v2];

== matlab function Dynamics/Jacobian/J(q) gen./J_v_3(q)/v2M_5 ==
  data: v1 input; M output; v2 input
function M = fcn(v1,v2)

M=[v1 v2];

== matlab function Dynamics/Jacobian/J(q) gen./J_v_4(q)/v2M_1 ==
  data: v1 input; M output; v2 input
function M = fcn(v1,v2)

M=[v1 v2];

== matlab function Dynamics/Jacobian/J(q) gen./J_v_4(q)/v2M_2 ==
  data: v1 input; M output; v2 input
function M = fcn(v1,v2)

M=[v1 v2];

== matlab function Dynamics/Jacobian/J(q) gen./J_v_4(q)/v2M_3 ==
  data: v1 input; M output; v2 input
function M = fcn(v1,v2)

M=[v1 v2];

== matlab function Dynamics/Jacobian/J(q) gen./J_v_4(q)/v2M_4 ==
  data: v1 input; M output; v2 input
function M = fcn(v1,v2)

M=[v1 v2];

== matlab function Dynamics/Jacobian/J(q) gen./J_v_4(q)/v2M_5 ==
  data: v1 input; M output; v2 input
function M = fcn(v1,v2)

M=[v1 v2];

== matlab function Dynamics/Jacobian/J(q) gen./J_v_5(q)/v2M_1 ==
  data: v1 input; M output; v2 input
function M = fcn(v1,v2)

M=[v1 v2];

== matlab function Dynamics/Jacobian/J(q) gen./J_v_5(q)/v2M_2 ==
  data: v1 input; M output; v2 input
function M = fcn(v1,v2)

M=[v1 v2];

== matlab function Dynamics/Jacobian/J(q) gen./J_v_5(q)/v2M_3 ==
  data: v1 input; M output; v2 input
function M = fcn(v1,v2)

M=[v1 v2];

== matlab function Dynamics/Jacobian/J(q) gen./J_v_5(q)/v2M_4 ==
  data: v1 input; M output; v2 input
function M = fcn(v1,v2)

M=[v1 v2];

== matlab function Dynamics/Jacobian/J(q) gen./J_v_5(q)/v2M_5 ==
  data: v1 input; M output; v2 input
function M = fcn(v1,v2)

M=[v1 v2];

== matlab function Dynamics/Jacobian/J(q) gen./MATLAB Function ==
  data: J_w1 input; J_q output; J_w2 input; J_w3 input; J_w4 input; J_w5 input; J_w6 input; J_v1 input; J_v2 input; J_v3 input; J_v4 input; J_v5 input; J_v6 input; R1 input; R2 input; R3 input; R4 input; R5 input; R6 input
function J_q = fcn(J_w1,J_w2,J_w3,J_w4,J_w5,J_w6,J_v1,J_v2,J_v3,J_v4,J_v5,J_v6,R1,R2,R3,R4,R5,R6)


J_q=[J_v1
     J_v2
     J_v3
     J_v4
     J_v5
     J_v6
     R1'*J_w1 zeros(3,5)
     R2'*J_w1 R2'*J_w2 zeros(3,4)
     R3'*J_w1 R3'*J_w2 R3'*J_w3 zeros(3,3)
     R4'*J_w1 R4'*J_w2 R4'*J_w3 R4'*J_w4 zeros(3,2)
     R5'*J_w1 R5'*J_w2 R5'*J_w3 R5'*J_w4 R5'*J_w5 zeros(3,1)
     R6'*J_w1 R6'*J_w2 R6'*J_w3 R6'*J_w4 R6'*J_w5 R6'*J_w6];
